simulink library "bcm"  (R2021b)
settings: Solver=VariableStepAuto  StartTime=0.0  StopTime=10.0  RelTol=1e-3
undefined symbols (not defined in the file or in its folder): ENUM_ANTITHEFT_ALARM, ENUM_ANTITHEFT_ARM, ENUM_ANTITHEFT_DISARM, ENUM_ANTITHEFT_WAIT, ENUM_GEARPOSNTOCAN_P, ENUM_PDKEYRAWLULOCK_INUNLOCK, ENUM_PDKEYRAWPS_INPS, ENUM_POWERSTA_ON, ENUM_POWERSTA_READY, ENUM_POWERSTA_STANDBY, ENUM_PWRSTASW_ON, ENUM_PWRSTASW_READY, ENUM_VEHICLETYPE_D21, ENUM_VEHICLETYPE_D31F25, ENUM_VEHICLETYPE_D31HAWD, ENUM_VEHICLETYPE_D31HRWD, ENUM_VEHICLETYPE_D31L24, FALSE, KBCM_ACCSwcPrsTmr_s, KBCM_ALMBrightnessDark_enum, KBCM_AmbBlue_enum, KBCM_AmbBreathT_ms, KBCM_AmbGreen_enum, KBCM_AmbMidPple_enum, KBCM_AmbRed_enum, KBCM_AmbTempCtrlEN_flg, KBCM_AmbTempT_s, KBCM_AmbWelModeENWait_s, KBCM_Antitheft_enum_ovrdflg, KBCM_Antitheft_enum_ovrdval, KBCM_APMDoorCtrlSta_flg_ovrdflg, KBCM_APMDoorCtrlSta_flg_ovrdval, KBCM_CmdKeepT_s, KBCM_CSWLightRstDebT_s, KBCM_CSWTurnLPRstT_s, KBCM_DelayTSW_flg, KBCM_DiagDRLOFF_flg, KBCM_DiagFLTC_mA, KBCM_DiagFMHT_s, KBCM_DiagFRTC_mA, KBCM_DiagRLTC_mA, KBCM_DiagRRTC_mA, KBCM_DrAPMRetryTimes_cnt, KBCM_DrOpenWdwOT_s, KBCM_DrOpenWdwReady_s, KBCM_ESSOffT_ms, KBCM_ESSOnT_ms, KBCM_FDCDKCReDetectT_K, KBCM_FDCDKCUSSFilterT_K, KBCM_HandleLampKeepT_s, KBCM_IVIRstHoldT_ms, KBCM_IVIRstTriggerT_ms, KBCM_ONDelayT_ms, KBCM_RAPSAbnFlashOFFT_ms, KBCM_RAPSAbnFlashONT_ms, KBCM_ReDetectT_K, KBCM_RightHandDriveEN_flg, KBCM_RLSLowSpdFilterT_s, KBCM_RmLampKeep_min, KBCM_RmLpKeyInT_s ... (+37)
libraries: simulink x447, $bdroot x11, hcu_lib x2
(part 12 of 13)

== stateflow chart bcm/BCM/BCM/CenterDoorLock/Chart ==
  settings: updateMethod=DISCRETE
  state CrashDetect [parallel]
    settings: executionOrder=7
    state OFF [commented out]
    state KeyON [commented out]
      state Initial [commented out]
        en:
        CrashDetd=0;
      state sCrash [commented out]
        en:CrashDetd=1;Unlockreq=1;
      note: 750 ms
      state Detect [commented out]
      Initial -> Detect [commented out] : [after(75,tick)]
      Detect -> sCrash [commented out] : [CrashOutputSts>0||....
          | (CrashInputFreq>4.1&&....
          | CrashInputFreq<4.2&&....
          | CrashInputDuty>16&&....
          | CrashInputDuty<17)]
    (default) -> CrashDetect.OFF [commented out]
    CrashDetect.OFF -> Initial [commented out] : [PwrSta>3]
    KeyON -> CrashDetect.OFF [commented out] : [PwrSta<=3]
    (default) -> (junction 1980)
    (junction 1980) -> (junction 1981) : [hasChanged(CrashDetd) && CrashDetd == TRUE]
    CrashDetect -> (junction 1980)
    (junction 1981) -> (junction 1979) : {Unlockreq=1;}
  state ChargingDoor [parallel]
    settings: executionOrder=1
    state ChargingDoorUnlock
      en:FrChargingDoorCtrl=0;
      RrChargingDoorCtrl=0;
      FuelDoorPos=0;
    state U2L
      en:FrChargingDoorCtrl=2;
      RrChargingDoorCtrl=2;
    note: 100ms
    note: 100ms
    state L2U
      en:FrChargingDoorCtrl=1;
      RrChargingDoorCtrl=1;
    state ChargingDoorLock
      en:FrChargingDoorCtrl=0;
      RrChargingDoorCtrl=0;
      FuelDoorPos=1;
    (default) -> (junction 1986)
    (junction 1986) -> (junction 1988) [order 2]
    (junction 1986) -> ChargingDoorUnlock [order 1] : [!EEP_FuelDoorPos]
    (junction 1988) -> ChargingDoorLock
    ChargingDoorUnlock -> U2L : [AntitheftSta==1||AntitheftSta==3]
    L2U -> ChargingDoorUnlock : [after(10,tick)]
    U2L -> ChargingDoorLock : [after(10,tick)]
    ChargingDoorLock -> L2U : [AntitheftSta==0||AntitheftSta==2]
  state IVICentralDoorLockSW [parallel]
    settings: executionOrder=3
    state Release
    state Press
    (default) -> IVICentralDoorLockSW.Press
    IVICentralDoorLockSW.Press -> IVICentralDoorLockSW.Release : [CDL_Unlock_Butt==0&&CDL_Lock_Butt==0]
    IVICentralDoorLockSW.Release -> (junction 1950) [order 1] : [CDL_Lock_Butt==1]
    (junction 1950) -> IVICentralDoorLockSW.Press [order 1] : [BCM_DoorLock_Sta]/{Main.eDUnlock;}
    (junction 1950) -> (junction 1951) [order 2]
    (junction 1951) -> IVICentralDoorLockSW.Press [order 1] : [AllDoorSW]/{Main.eDUnlock;}
    (junction 1951) -> (junction 1952) [order 2]
    (junction 1952) -> IVICentralDoorLockSW.Press [order 1] : [CrashDetd==1]{Main.eDUnlock;}
    (junction 1952) -> (junction 1953) [order 2]
    (junction 1953) -> IVICentralDoorLockSW.Press : {Main.eCTDLock;}
    IVICentralDoorLockSW.Release -> IVICentralDoorLockSW.Press [order 2] : [CDL_Unlock_Butt==1]{Main.eDUnlock;}
  state ATLockCtrl [parallel]
    settings: executionOrder=4
    state LockSend
      en:
      fUnlockSingle=1;
    state NoCommand
    state UnlockSend
      en:fUnlockSingle=0;
    (default) -> NoCommand : {fUnlockSingle=VINP_FlashfUnlockSingle_flg;}
    NoCommand -> (junction 1862) [order 2] : [ATLockCtrl==1]
    (junction 1862) -> LockSend [order 1] : [CrashDetd==1]
    (junction 1862) -> (junction 1865) [order 2] : {Main.eDLock;}
    (junction 1865) -> LockSend [order 1] : [LockSetting]
    (junction 1865) -> (junction 1867) [order 2]
    (junction 1867) -> LockSend
    LockSend -> NoCommand : [ATLockCtrl!=1]
    NoCommand -> (junction 1870) [order 1] : [ATLockCtrl==2....
        | ||....
        | VBCM_AutoUnlockReq_flg]
    (junction 1870) -> UnlockSend [order 1] : [LockSetting==0||fUnlockSingle==0]/{Main.eDUnlock;}
    (junction 1870) -> (junction 1872) [order 2]
    (junction 1872) -> UnlockSend : /{Main.eSUnlock;}
    UnlockSend -> NoCommand : [ATLockCtrl!=2 && !VBCM_AutoUnlockReq_flg]
  state CentralDoorLockSW [parallel]
    settings: executionOrder=2
    state Release
    state Press
    (default) -> CentralDoorLockSW.Press
    CentralDoorLockSW.Press -> CentralDoorLockSW.Release : [!CentralDoorLockSW]
    CentralDoorLockSW.Release -> (junction 1817) : [CentralDoorLockSW]
    (junction 1817) -> CentralDoorLockSW.Press [order 1] : [BCM_DoorLock_Sta]/{Main.eDUnlock;}
    (junction 1817) -> (junction 1821) [order 2]
    (junction 1821) -> CentralDoorLockSW.Press [order 1] : [AllDoorSW]/{Main.eDUnlock;}
    (junction 1821) -> (junction 1824) [order 2]
    (junction 1824) -> CentralDoorLockSW.Press [order 1] : [CrashDetd==1]{Main.eDUnlock;}
    (junction 1824) -> (junction 1827) [order 2]
    (junction 1827) -> CentralDoorLockSW.Press : {Main.eCTDLock;}
  state AutoFoldforHandle [parallel]
    settings: executionOrder=10
    state sStop
    state sMoving
    (default) -> sStop
    sMoving -> sStop : [VehSpeed <= 0]
    sStop -> (junction 2026) : [VehSpeed >= 10 && VehSpeed < 256]
    (junction 2026) -> sMoving [order 1] : [!CrashDetd && ...
        | (!VINP_FLHandleClose_flg || !VINP_FRHandleClose_flg || ....
        |  !VINP_RLHandleClose_flg || !VINP_RRHandleClose_flg)]
        | {VBCM_FDHandleCmd_enum = 3;
        |  LHandleLampCtrl = 1;
        |  RHandleLampCtrl = 1;}
    (junction 2026) -> (junction 2027) [order 2]
    (junction 2027) -> sMoving
  state LED [parallel]
    settings: executionOrder=6
    state OFF
      en:DoorLockIND=0;
    state ON
      en:DoorLockIND=1;
    note: 10 sec
    state HoldON
      en:DoorLockIND=1;
    (default) -> LED.OFF
    ON -> LED.OFF [order 1] : [BCM_DoorLock_Sta==0]
    LED.OFF -> ON [order 1] : [PwrSta>3&&BCM_DoorLock_Sta==1]
    HoldON -> LED.OFF [order 1] : [after(1000,tick)||BCM_DoorLock_Sta==0]
    LED.OFF -> HoldON [order 2] : eResetLED[BCM_DoorLock_Sta==1]
    HoldON -> ON [order 2] : [PwrSta>3]
    ON -> HoldON [order 2] : [PwrSta<=3]
    HoldON -> HoldON [order 3] : eResetLED
  state Main [parallel]
    settings: executionOrder=5
    note: 350 ms
    state WaitForReverse
      en:CTDCtrl=0;
    state StandBy
      en:CTDCtrl=0;
    state DoorLock
      en:CTDCtrl=3;
    note: 100 ms
    state DrDoorUnlock
      en:CTDCtrl=1;
      fVIGHandle=0;
    note: Unlockreq
    state DoorUnlock
      en:CTDCtrl=2;
      fVIGHandle=0;
      ex:Unlockreq=0;
    (default) -> Main.StandBy
    Main.StandBy -> DoorLock [order 1] : eDLock
    DoorLock -> WaitForReverse [order 1] : [after(35,tick)]/{LED.eResetLED;}
    DoorLock -> WaitForReverse [order 2] : [Unlockreq]/{LED.eResetLED;}
    Main.StandBy -> DoorLock [order 5] : eCTDLock{fVIGHandle=1;}
    WaitForReverse -> Main.StandBy : [after(10,tick)]
    Main.StandBy -> DrDoorUnlock [order 2] : eSUnlock
    DrDoorUnlock -> WaitForReverse [order 1] : [after(35,tick)]
    DrDoorUnlock -> DoorUnlock [order 2] : eDUnlock
    DrDoorUnlock -> DoorUnlock [order 3] : [Unlockreq]
    DoorUnlock -> WaitForReverse : [after(35,tick)]
    Main.StandBy -> DoorUnlock [order 3] : eDUnlock
    Main.StandBy -> DoorUnlock [order 4] : [Unlockreq]
  state LHandleLampPowerCtrlforHandle [parallel]
    settings: executionOrder=12
    state sKeep
      en:
      VBCM_FDLHandleLampCmd_flg = 1;
    state sStandBy
      en:
      VBCM_FDLHandleLampCmd_flg = 0;
      LHandleLampCtrl = 0;
    LHandleLampPowerCtrlforHandle -> LHandleLampPowerCtrlforHandle.sKeep : [hasChanged(VBCM_FDHandleCmd_enum) && ...
        | (VBCM_FDHandleCmd_enum == 1 || ...
        |  VBCM_FDHandleCmd_enum == 2)]
    LHandleLampPowerCtrlforHandle.sKeep -> LHandleLampPowerCtrlforHandle.sStandBy : [after (KBCM_HandleLampKeepT_s, tick) || ...
        | (LHandleLampCtrl && ...
        |  VINP_FLHandleClose_flg)]
    (default) -> LHandleLampPowerCtrlforHandle.sStandBy
  state DoorOpenDetectforHandle [parallel]
    settings: executionOrder=8
    state sDrDoorOpenDet [parallel]
      settings: executionOrder=1
      (default) -> (junction 2039)
      sDrDoorOpenDet -> (junction 2038) : [hasChanged(VINP_DrDoorSW_flg) && VINP_DrDoorSW_flg]
      (junction 2038) -> (junction 2039) : [VehSpeed <= 0 && VINP_FLHandleClose_flg]
          | {VBCM_FDHandleCmd_enum = 1;
          |  LHandleLampCtrl = 0;}
    state sPsDoorOpenDet [parallel]
      settings: executionOrder=2
      (default) -> (junction 2045)
      (junction 2044) -> (junction 2045) : [VehSpeed <= 0 && ...
          | (VINP_FLHandleClose_flg || VINP_FRHandleClose_flg)]
          | {VBCM_FDHandleCmd_enum = 2;
          |  RHandleLampCtrl = 0;}
      sPsDoorOpenDet -> (junction 2044) : [hasChanged(VINP_PsDoorSW_flg) && VINP_PsDoorSW_flg]
    state sRLDoorOpenDet [parallel]
      settings: executionOrder=3
      (default) -> (junction 2051)
      sRLDoorOpenDet -> (junction 2050) : [hasChanged(VINP_RLDoorSW_flg) && VINP_RLDoorSW_flg]
      (junction 2050) -> (junction 2051) : [VehSpeed <= 0 && ...
          | (VINP_FLHandleClose_flg || VINP_RLHandleClose_flg)]
          | {VBCM_FDHandleCmd_enum = 2;
          |  RHandleLampCtrl = 0;}
    state sRRDoorOpenDet [parallel]
      settings: executionOrder=4
      (default) -> (junction 2057)
      sRRDoorOpenDet -> (junction 2056) : [hasChanged(VINP_RRDoorSW_flg) && VINP_RRDoorSW_flg]
      (junction 2056) -> (junction 2057) : [VehSpeed <= 0 && ...
          | (VINP_FLHandleClose_flg || VINP_RRHandleClose_flg)]
          | {VBCM_FDHandleCmd_enum = 2;
          |  RHandleLampCtrl = 0;}
  state AutoLock [parallel]
    settings: executionOrder=14
    state StandBy
      en:
      VBCM_AutoUnlockReq_flg = 0;
    state AutoLock
      en:
      Main.eDLock;
      VBCM_AutoLockDisable_flg = 1;
    state AutoUnlock
      en:
      VBCM_AutoUnlockReq_flg = 1;
      VBCM_AutoLockDisable_flg = 0;
    state AutoLockENRst
      en:
      VBCM_AutoLockDisable_flg = 0;
    (default) -> AutoLock.StandBy
    AutoLock.StandBy -> AutoLock.AutoLock [order 3] : [AirBagFailCmd==0 && CrashDetd==0 && VehSpeed>=10 && VBCM_AutoLockSta_flg && !VBCM_AutoLockDisable_flg]
    AutoLock.AutoLock -> AutoLock.StandBy
    AutoLock.StandBy -> AutoUnlock [order 1] : [VBCM_AutoUnlockSta_flg && ShiftGearPosnBuf != 0 && VTQD_ShiftGearPosn_enum == 0]
    AutoUnlock -> AutoLock.StandBy
    AutoLock.StandBy -> AutoLockENRst [order 2] : [(hasChanged(AllDoorSW) && AllDoorSW == 1)....
        | ||....
        | (PwrStaBuf == 4 || PwrStaBuf == 5) && (PwrSta >= 0 && PwrSta <= 3)....
        | ||....
        | (hasChanged(VBCM_AutoLockSta_flg) && VBCM_AutoLockSta_flg)]
    AutoLockENRst -> AutoLock.StandBy
  state RHandleLampPowerCtrlforHandle [parallel]
    settings: executionOrder=13
    state sKeep
      en:
      VBCM_FDRHandleLampCmd_flg = 1;
    state sStandBy
      en:
      VBCM_FDRHandleLampCmd_flg = 0;
      RHandleLampCtrl = 0;
    RHandleLampPowerCtrlforHandle -> RHandleLampPowerCtrlforHandle.sKeep : [hasChanged(VBCM_FDHandleCmd_enum) && ....
        | VBCM_FDHandleCmd_enum == 2]
    RHandleLampPowerCtrlforHandle.sKeep -> RHandleLampPowerCtrlforHandle.sStandBy : [after (KBCM_HandleLampKeepT_s, tick) || ...
        | (RHandleLampCtrl && ...
        |  VINP_FRHandleClose_flg &&....
        |  VINP_RLHandleClose_flg &&....
        |  VINP_RRHandleClose_flg)]
    (default) -> RHandleLampPowerCtrlforHandle.sStandBy
  state CmdReset [parallel]
    settings: executionOrder=11
    state sKeep
    state sStandBy
      en:
      VBCM_FDHandleCmd_enum = 0;
    CmdReset -> CmdReset.sKeep : [hasChanged(VBCM_FDHandleCmd_enum) && ...
        | VBCM_FDHandleCmd_enum > 0]
    CmdReset.sKeep -> CmdReset.sStandBy : [after (KBCM_CmdKeepT_s, tick)]
    (default) -> CmdReset.sStandBy
  state CTDDoorCtrlforHandle [parallel]
    settings: executionOrder=9
    (default) -> (junction 2009)
    (junction 2008) -> (junction 2009) [order 1] : [VehSpeed <= 0 && CTDCtrl == 1]
        | {VBCM_FDHandleCmd_enum = CTDCtrl;
        |  LHandleLampCtrl = 0;}
    CTDDoorCtrlforHandle -> (junction 2008) : [hasChanged(CTDCtrl) && CTDCtrl > 0]
    (junction 2008) -> (junction 2010) [order 2]
    (junction 2010) -> (junction 2011) [order 1] : [VehSpeed <= 0 && CTDCtrl == 2]
        | {VBCM_FDHandleCmd_enum = CTDCtrl;
        |  LHandleLampCtrl = 0;
        |  RHandleLampCtrl = 0;}
    (junction 2010) -> (junction 2012) [order 2] : [VehSpeed <= 0 && CTDCtrl == 3]
        | {VBCM_FDHandleCmd_enum = CTDCtrl;
        |  LHandleLampCtrl = 1;
        |  RHandleLampCtrl = 1;}
  data: AntitheftSta input uint8 [..3]; FrChargingDoorCtrl output uint8 [0..2]; RrChargingDoorCtrl output uint8 [0..2]; AllDoorSW input boolean; PwrSta input uint8 [0..5]; CentralDoorLockSW input boolean; BCM_DoorLock_Sta input boolean; CTDCtrl output uint8 [0..3]; DoorLockIND output boolean; ATLockCtrl input uint8 [0..2]; AirBagFailCmd input boolean; VehSpeed input; fVIGHandle output boolean; CDL_Unlock_Butt input boolean; CDL_Lock_Butt input boolean; Unlockreq local boolean; CrashDetd input boolean; FuelDoorPos output; EEP_FuelDoorPos input; fUnlockSingle output boolean; VINP_FlashfUnlockSingle_flg input; KBCM_CmdKeepT_s input; KBCM_HandleLampKeepT_s input; VINP_DrDoorSW_flg input; VINP_FLHandleClose_flg input; VINP_FRHandleClose_flg input; VINP_PsDoorSW_flg input; VINP_RLDoorSW_flg input; VINP_RLHandleClose_flg input; VINP_RRDoorSW_flg input; VINP_RRHandleClose_flg input; VBCM_FDLHandleLampCmd_flg output boolean; VBCM_FDRHandleLampCmd_flg output boolean; LHandleLampCtrl local boolean; RHandleLampCtrl local boolean; VBCM_FDHandleCmd_enum output uint8; LockSetting input =0; PwrStaBuf input; ShiftGearPosnBuf input; VBCM_AutoLockSta_flg input; VBCM_AutoUnlockSta_flg input; VTQD_ShiftGearPosn_enum input; VBCM_AutoLockDisable_flg local boolean; VBCM_AutoUnlockReq_flg local boolean; TRUE parameter
  events: eResetLED local FUNCTION_CALL_EVENT; eDLock local FUNCTION_CALL_EVENT; eDUnlock local FUNCTION_CALL_EVENT; eSUnlock local FUNCTION_CALL_EVENT; eCTDLock local FUNCTION_CALL_EVENT

== stateflow chart bcm/BCM/BCM/Dimmer/Chart ==
  settings: sampleTime=StepSize
  state CANDimmerCMD [parallel]
    settings: executionOrder=1
    state sWait
    (default) -> sWait
    (junction 1680) -> sWait : [MFRD_N_Bright_Req<=100&&IVI_Status]/{Dimmer=20+MFRD_N_Bright_Req*0.8}
    (junction 1677) -> (junction 1680) [order 1]
    (junction 1677) -> sWait [order 2]
    (junction 1609) -> (junction 1677)
    sWait -> (junction 1609) : [after(20,tick)]
  state sDimmer_EN [parallel]
    settings: executionOrder=2  description=This state models the modes of a door sensor and implements logic to respond when that sensor is producing a signal.
    state sOFF
      en:DimmerEN=0;
    state sON
      en:DimmerEN=1;
    (default) -> sOFF
      settings: description=On the first sample call the door mode is set to active.
    sON -> sOFF : [!PLamp||IVI_Night_Mode_Sta]
    sOFF -> sON : [PLamp&&!IVI_Night_Mode_Sta]
  data: IVI_Status input boolean; IVI_Night_Mode_Sta input boolean; Dimmer output single =0; DimmerEN output boolean; PLamp input boolean; MFRD_N_Bright_Req input =0
  data IVI_Night_Mode_Sta settings: description=Min=0, Max=2047, Engineering Unit = km/h, Offset=0 km/h, Resolution= 0.125 km/h per bit, >2047 = Invalid (bit 12 = 1)
  data Dimmer settings: description=|
      | Bcm Buzzer output results.
      | 0 = None Buzzer
      | 1 = Turn signal Buzzer
      | 2 = Key Reminder Buzzer
      | 3 = Seat Belt Buzzer
      | 4 = Light Monitor Buzzer

== stateflow chart bcm/BCM/BCM/ExteriorLight/Chart ==
  settings: updateMethod=DISCRETE
  state FollowMeSW [parallel]
    settings: executionOrder=2
    state Disabled
    state Enabled
    (default) -> Disabled
    Disabled -> Enabled : [FDC_BCM_FollowMeENFun_Sta==1]
    Enabled -> (junction 2763) [order 2] : [(VBCM_PwrStaBuf_enum==4 || VBCM_PwrStaBuf_enum==5) &&....
        | (VPMM_PwrSta_enum==1 || VPMM_PwrSta_enum==2)]
        | {AutoCut.eFollow;}
    (junction 2763) -> (junction 2765)
    (junction 2755) -> Disabled [order 1] : [VBCM_FollowMe_flg==1]
        | {AutoCut.eFollow;}
    Enabled -> (junction 2755) [order 1] : [FDC_BCM_FollowMeENFun_Sta==0]
    (junction 2755) -> (junction 2758) [order 2]
    (junction 2765) -> Enabled
    (junction 2758) -> Disabled
  state RFogLamp [parallel]
    settings: executionOrder=1
    state sON
      en:VBCM_RrFogLamp_flg=1;
    state sOFF
      en:VBCM_RrFogLamp_flg=0;
    (default) -> RFogLamp.sOFF
    RFogLamp.sOFF -> RFogLamp.sON : [VPMM_PwrSta_enum>3&&....
        | VINP_RFogLampSW_flg==1&&....
        | VBCM_LBeam_flg==1]
    RFogLamp.sON -> RFogLamp.sOFF : [VPMM_PwrSta_enum<=3||....
        | VINP_RFogLampSW_flg==0||....
        | VBCM_LBeam_flg==0]
  state DRL [parallel]
    settings: executionOrder=3
    state sOFF
      en:VBCM_LDRL_flg=0;
      VBCM_RDRL_flg=0;
    state DRL_Opearting
      state sDebounce
      state sON
        en:VBCM_LDRL_flg=1;
        VBCM_RDRL_flg=1;
      note: 300 ms
      state TurnLeft
        en:VBCM_LDRL_flg=0;
        VBCM_RDRL_flg=1;
      state TurnRight
        en:VBCM_LDRL_flg=1;
        VBCM_RDRL_flg=0;
      sDebounce -> (junction 2687) : [after(30,tick)]
      (junction 2687) -> DRL.DRL_Opearting.sON [order 1] : [VBCM_OutMode_enum==0]
      (junction 2687) -> (junction 2689) [order 2]
      DRL.DRL_Opearting.sON -> TurnLeft [order 1] : [VBCM_OutMode_enum==1]
      TurnLeft -> DRL.DRL_Opearting.sON [order 1] : [VBCM_OutMode_enum==0]
      TurnRight -> DRL.DRL_Opearting.sON [order 2] : [VBCM_OutMode_enum==0]
      DRL.DRL_Opearting.sON -> TurnRight [order 2] : [VBCM_OutMode_enum==2]
      (junction 2689) -> TurnLeft [order 1] : [VBCM_OutMode_enum==1]
      (junction 2689) -> (junction 2701) [order 2]
      TurnRight -> TurnLeft [order 1] : [VBCM_OutMode_enum==1]
      TurnLeft -> TurnRight [order 2] : [VBCM_OutMode_enum==2]
      (junction 2701) -> TurnRight
    (default) -> DRL.sOFF
    DRL.sOFF -> sDebounce : [VBCM_DiagDRLOFF_flg==0 &&...
        | VPMM_PwrSta_enum==ENUM_POWERSTA_READY &&...
        | (VTQD_ShiftGearPosn_enum != ENUM_GEARPOSNTOCAN_P || VINP_HeadLampSW_enum==0) &&...
        | !VBCM_PosLamp_flg &&...
        | VBCM_OutMode_enum < 3]
    DRL_Opearting -> DRL.sOFF : [VBCM_DiagDRLOFF_flg==1 ||...
        | VPMM_PwrSta_enum!=ENUM_POWERSTA_READY ||...
        | (VTQD_ShiftGearPosn_enum == ENUM_GEARPOSNTOCAN_P && VINP_HeadLampSW_enum!=0) ||...
        | VBCM_PosLamp_flg ||...
        | VBCM_OutMode_enum >= 3]
  state sBrakeLamp [parallel]
    settings: executionOrder=4
    state sON
      en:VBCM_BrakeLamp_flg=1;
    state sOFF
      en:VBCM_BrakeLamp_flg=0;
    (default) -> sBrakeLamp.sOFF
    sBrakeLamp.sOFF -> sBrakeLamp.sON : [VINP_BrakeSWGPIO_flg==1 || VTQD_ReBrakeLPReq_flg==1 || VINP_ActBrkLampSta_flg==1]
    sBrakeLamp.sON -> sBrakeLamp.sOFF : [VINP_BrakeSWGPIO_flg==0 && VTQD_ReBrakeLPReq_flg==0 && VINP_ActBrkLampSta_flg==0]
  state sReverseLamp [parallel]
    settings: executionOrder=5
    state sON
      en:VBCM_ReverseLamp_flg=1;
    state sOFF
      en:VBCM_ReverseLamp_flg=0;
    (default) -> sReverseLamp.sOFF
    sReverseLamp.sOFF -> sReverseLamp.sON : [VPMM_PwrSta_enum>3&&VTQD_ShiftGearPosn_enum==7]
    sReverseLamp.sON -> sReverseLamp.sOFF : [VPMM_PwrSta_enum<=3||VTQD_ShiftGearPosn_enum!=7]
  state sATCtrl [parallel]
    settings: executionOrder=6
    state StandBy
    state Lock
      en:send(AutoCut.eLock);
    state Unlock
      en:send(AutoCut.eUnlock);
    (default) -> StandBy
    StandBy -> Lock [order 1] : [VBCM_ATCtrl_enum==1]
    Lock -> StandBy : [VBCM_ATCtrl_enum!=1]
    StandBy -> sATCtrl.Unlock [order 2] : [VBCM_ATCtrl_enum==2]
    sATCtrl.Unlock -> StandBy : [VBCM_ATCtrl_enum!=2]
  state PositionLamp [parallel]
    settings: executionOrder=11
    state sPositionLamp
      en:VBCM_PosLamp_flg=1;
    state sOFF
      en:VBCM_PosLamp_flg=0;
    (default) -> PositionLamp.sOFF
    (junction 2636) -> sPositionLamp [order 1] : [VINP_HeadLampSW_enum==1||VINP_HeadLampSW_enum==2]
    PositionLamp.sOFF -> (junction 2636) [order 1] : [!VBCM_AutoCut_flg]
    (junction 2636) -> (junction 2637) [order 2]
    (junction 2637) -> sPositionLamp [order 1] : [VPMM_PwrSta_enum > 3 &&....
        | VINP_HeadLampSW_enum == 0 &&....
        | VINP_RLSLampSta_flg]
    (junction 2637) -> (junction 2638) [order 2]
    (junction 2638) -> sPositionLamp : [VBCM_FollowMe_flg]
    PositionLamp.sOFF -> sPositionLamp [order 2] : [VBCM_showupEN_flg && VBCM_showup_flg]
    (junction 2639) -> PositionLamp.sOFF : [!VBCM_FollowMe_flg &&....
        | (VINP_HeadLampSW_enum == 3 ||....
        | (VINP_HeadLampSW_enum == 0 &&....
        | (VPMM_PwrSta_enum <= 3 || !VINP_RLSLampSta_flg)))]
    (junction 2640) -> (junction 2639) [order 2]
    (junction 2640) -> PositionLamp.sOFF [order 1] : [VBCM_AutoCut_flg]
    sPositionLamp -> (junction 2640) : [!VBCM_showupEN_flg || !VBCM_showup_flg]
  state AutoCut [parallel]
    settings: executionOrder=12
    state FollowMeHome
      en:
      VBCM_FollowMe_flg=1;
      VBCM_AutoCut_flg=0;
      VBCM_showup_flg=0;
      ex:
      VBCM_FollowMe_flg=0;
    state Normal
      state sNormal
        en:VBCM_AutoCut_flg=0;
        VBCM_showup_flg=0;
      state AutoCutDetect
      note: 40 sec
      state Unlock
        en:VBCM_AutoCut_flg=1;
        VBCM_showup_flg=1;
        note: 30 sec
      state AutoCut
        en:VBCM_AutoCut_flg=1;
        VBCM_showup_flg=0;
        VBCM_FollowMe_flg=0;
      sNormal -> AutoCutDetect : [VPMM_PwrSta_enum<=3&&(VINP_HeadLampSW_enum!=3)]
      (junction 2665) -> sNormal : [VPMM_PwrSta_enum>3||VINP_HeadLampSW_enum==3]
      AutoCutDetect -> (junction 2665) [order 1]
      AutoCut.Normal.AutoCut -> (junction 2665)
      AutoCutDetect -> AutoCut.Normal.AutoCut [order 2] : eLock
      AutoCutDetect -> AutoCut.Normal.AutoCut [order 3] : [after(4000,tick)]
      AutoCut.Normal.Unlock -> sNormal [order 2] : [VPMM_PwrSta_enum>3]
      (default) -> AutoCut.Normal.AutoCut
      AutoCut.Normal.Unlock -> AutoCut.Normal.AutoCut [order 1] : eLock
      AutoCut.Normal.Unlock -> AutoCut.Normal.AutoCut [order 3] : [after(3000,tick)]
      Normal -> AutoCut.Normal.Unlock [order 1] : eUnlock[VPMM_PwrSta_enum<=3]
    note: 4000
    note: 40 sec
    (default) -> Normal
    Normal -> FollowMeHome [order 1] : eFollow[VPMM_PwrSta_enum<=3]
    FollowMeHome -> sNormal [order 2] : eFollow
    FollowMeHome -> sNormal [order 3] : [VPMM_PwrSta_enum>3]
    FollowMeHome -> (junction 2717) [order 1] : [after(VBCM_DiagFMHT_s,tick)]
    (junction 2717) -> sNormal [order 1] : [VPMM_PwrSta_enum>3||...
        |  VINP_HeadLampSW_enum==3]
    (junction 2717) -> (junction 2719) [order 2]
    (junction 2719) -> AutoCut.Normal.AutoCut
  state LowBeam [parallel]
    settings: executionOrder=8
    state sLBeam
      en:VBCM_LBeam_flg=1;
    state sOFF
      en:VBCM_LBeam_flg=0;
    (default) -> LowBeam.sOFF
    (junction 2417) -> sLBeam [order 1] : [VBCM_HBeam_flg]
    LowBeam.sOFF -> (junction 2417) [order 1] : [!VBCM_AutoCut_flg]
    (junction 2417) -> (junction 2418) [order 2]
    (junction 2418) -> sLBeam [order 1] : [VINP_HeadLampSW_enum==2]
    (junction 2418) -> (junction 2419) [order 2]
    (junction 2419) -> sLBeam [order 1] : [VPMM_PwrSta_enum > VBCM_HLBeamENPwrSta_enum &&....
        | VINP_HeadLampSW_enum == 0 &&....
        | VINP_RLSLampSta_flg]
    (junction 2419) -> (junction 2420) [order 2]
    (junction 2420) -> sLBeam : [VBCM_FollowMe_flg]
    LowBeam.sOFF -> sLBeam [order 2] : [VBCM_showupEN_flg && VBCM_showup_flg]
    (junction 2421) -> LowBeam.sOFF [order 1] : [VBCM_AutoCut_flg]
    sLBeam -> (junction 2421) : [!VBCM_showupEN_flg || !VBCM_showup_flg]
    (junction 2421) -> (junction 2422) [order 2]
    (junction 2422) -> LowBeam.sOFF : [!VBCM_FollowMe_flg &&....
        | !VBCM_HBeam_flg &&....
        | VINP_HeadLampSW_enum != 2 &&....
        | (VINP_HeadLampSW_enum!=0 ||....
        | !VINP_RLSLampSta_flg ||....
        | VPMM_PwrSta_enum <= VBCM_HLBeamENPwrSta_enum)]
  state HighBeam [parallel]
    settings: executionOrder=7
    state sOFF
      en:VBCM_HBeam_flg=0;
    state sHBeam
      en:VBCM_HBeam_flg=1;
    (default) -> HighBeam.sOFF
    HighBeam.sOFF -> (junction 2455) : [!VBCM_AutoCut_flg]
    (junction 2455) -> HighBeam.sHBeam [order 1] : [VINP_CSWPassSWSta_flg]
    (junction 2455) -> (junction 2456) [order 2]
    (junction 2456) -> (junction 2457) : [VINP_CSWDimSw_flg]
    (junction 2457) -> HighBeam.sHBeam [order 1] : [VINP_HeadLampSW_enum==2]
    (junction 2457) -> (junction 2458) [order 2]
    (junction 2458) -> HighBeam.sHBeam : [VINP_HeadLampSW_enum == 0 &&....
        | VINP_RLSLampSta_flg == 1 &&....
        | VINP_ForceLowBeam_enum == 0 &&....
        | VPMM_PwrSta_enum > VBCM_HLBeamENPwrSta_enum &&....
        | VBCM_AutoHLB_flg]
    HighBeam.sHBeam -> HighBeam.sOFF [order 1] : [VBCM_AutoCut_flg]
    HighBeam.sHBeam -> (junction 2459) [order 2] : [!VINP_CSWPassSWSta_flg]
    (junction 2459) -> HighBeam.sOFF [order 1] : [!VINP_CSWDimSw_flg]
    (junction 2459) -> (junction 2605) [order 2]
    (junction 2605) -> (junction 2460) : [VINP_HeadLampSW_enum!=2]
    (junction 2460) -> HighBeam.sOFF [order 1] : [VINP_HeadLampSW_enum!=0]
    (junction 2460) -> (junction 2462) [order 2]
    (junction 2462) -> HighBeam.sOFF [order 1] : [VINP_RLSLampSta_flg==0 || VPMM_PwrSta_enum <= VBCM_HLBeamENPwrSta_enum]
    (junction 2462) -> (junction 2463) [order 2]
    (junction 2463) -> HighBeam.sOFF : [VINP_ForceLowBeam_enum==1||!VBCM_AutoHLB_flg]
  state AutoHLB [parallel]
    settings: executionOrder=13
    state AutoON
      on after(KBCM_ONDelayT_ms, tick):
      VBCM_AutoHLB_flg = TRUE;
    state AutoOFF
      en:
      VBCM_AutoHLB_flg = FALSE;
    (default) -> AutoOFF
    AutoOFF -> AutoON : [VINP_METERKPHCalcu_kph >= 30]
    AutoON -> AutoOFF : [VINP_METERKPHCalcu_kph <= 25]
  state RBSD_CTRL [parallel]
    settings: executionOrder=10
    state OFF
      en:VBCM_RBSD_flg=0;
    state FlashOFF
      en:VBCM_RBSD_flg=0;
    state ON
      en:VBCM_RBSD_flg=1;
    (default) -> RBSD_CTRL.OFF
    RBSD_CTRL.FlashOFF -> RBSD_CTRL.OFF [order 1] : [VINP_SRRBSDWarnR_enum==0 && VINP_SRRODAWarnR_enum==0]
    RBSD_CTRL.ON -> RBSD_CTRL.FlashOFF [order 2] : [after(13,tick)&&(VINP_SRRBSDWarnR_enum==2||VINP_SRRODAWarnR_enum==2)]
    RBSD_CTRL.FlashOFF -> RBSD_CTRL.ON [order 2] : [after(12,tick)]
    RBSD_CTRL.ON -> RBSD_CTRL.OFF [order 1] : [VINP_SRRBSDWarnR_enum==0 && VINP_SRRODAWarnR_enum==0]
    RBSD_CTRL.OFF -> RBSD_CTRL.ON : [VINP_SRRBSDWarnR_enum>0 || VINP_SRRODAWarnR_enum>0]
  state LBSD_CTRL [parallel]
    settings: executionOrder=9
    state OFF
      en:VBCM_LBSD_flg=0;
    state FlashOFF
      en:VBCM_LBSD_flg=0;
    state ON
      en:VBCM_LBSD_flg=1;
    (default) -> LBSD_CTRL.OFF
    LBSD_CTRL.FlashOFF -> LBSD_CTRL.OFF [order 1] : [VINP_SRRBSDWarnL_enum==0 && VINP_SRRODAWarnL_enum==0]
    LBSD_CTRL.ON -> LBSD_CTRL.FlashOFF [order 2] : [after(13,tick)&&(VINP_SRRBSDWarnL_enum==2||VINP_SRRODAWarnL_enum==2)]
    LBSD_CTRL.FlashOFF -> LBSD_CTRL.ON [order 2] : [after(12,tick)]
    LBSD_CTRL.ON -> LBSD_CTRL.OFF [order 1] : [VINP_SRRBSDWarnL_enum==0 && VINP_SRRODAWarnL_enum==0]
    LBSD_CTRL.OFF -> LBSD_CTRL.ON : [VINP_SRRBSDWarnL_enum>0 || VINP_SRRODAWarnL_enum>0]
  state HighBeam_ADB [parallel]
    settings: executionOrder=14
    state sHBeam
      en:VBCM_HBeamADB_flg=1;
    state sOFF
      en:VBCM_HBeamADB_flg=0;
    (default) -> HighBeam_ADB.sOFF
    (junction 2723) -> HighBeam_ADB.sHBeam [order 1] : [VINP_CSWPassSWSta_flg]
    HighBeam_ADB.sOFF -> (junction 2723) : [!VBCM_AutoCut_flg]
    (junction 2723) -> (junction 2724) [order 2]
    (junction 2725) -> HighBeam_ADB.sHBeam [order 1] : [VINP_HeadLampSW_enum==2]
    (junction 2724) -> (junction 2725) : [VINP_CSWDimSw_flg]
    (junction 2725) -> (junction 2726) [order 2]
    (junction 2726) -> HighBeam_ADB.sHBeam : [VINP_HeadLampSW_enum == 0 &&....
        | VINP_RLSLampSta_flg == 1 &&....
        | VPMM_PwrSta_enum > VBCM_HLBeamENPwrSta_enum]
    HighBeam_ADB.sHBeam -> HighBeam_ADB.sOFF [order 1] : [VBCM_AutoCut_flg]
    (junction 2727) -> HighBeam_ADB.sOFF [order 1] : [!VINP_CSWDimSw_flg]
    HighBeam_ADB.sHBeam -> (junction 2727) [order 2] : [!VINP_CSWPassSWSta_flg]
    (junction 2727) -> (junction 2729) [order 2]
    (junction 2728) -> HighBeam_ADB.sOFF [order 1] : [VINP_HeadLampSW_enum!=0]
    (junction 2729) -> (junction 2728) : [VINP_HeadLampSW_enum!=2]
    (junction 2728) -> (junction 2730) [order 2]
    (junction 2730) -> HighBeam_ADB.sOFF : [VINP_RLSLampSta_flg == 0 ||....
        | VPMM_PwrSta_enum <= VBCM_HLBeamENPwrSta_enum]
  data: VPMM_PwrSta_enum input uint8 [0..5]; VBCM_PwrStaBuf_enum input uint8; VINP_HeadLampSW_enum input uint8 [0..3]; VINP_RFogLampSW_flg input boolean; VINP_BrakeSWGPIO_flg input boolean; VINP_CSWDimSw_flg input boolean; VINP_CSWPassSWSta_flg input boolean; VTQD_ShiftGearPosn_enum input uint8 [0..15]; VBCM_PosLamp_flg output boolean; VBCM_LBeam_flg output boolean; VBCM_HBeam_flg output boolean; VBCM_RrFogLamp_flg output boolean; VBCM_BrakeLamp_flg output boolean; VBCM_ReverseLamp_flg output boolean; VBCM_OutMode_enum input uint8 [0..15]; VBCM_AutoCut_flg local boolean; VBCM_LDRL_flg output boolean; VBCM_RDRL_flg output boolean; VBCM_ATCtrl_enum input uint8 [0..2]; VINP_RLSLampSta_flg input boolean; VINP_ActBrkLampSta_flg input boolean; VINP_SRRODAWarnR_enum input; VINP_SRRODAWarnL_enum input; VINP_SRRBSDWarnR_enum input; VINP_SRRBSDWarnL_enum input; VINP_ForceLowBeam_enum input uint8; VTQD_ReBrakeLPReq_flg input; VBCM_LBSD_flg output boolean; VBCM_RBSD_flg output boolean; VBCM_DiagDRLOFF_flg input; VBCM_DiagFMHT_s input; ENUM_GEARPOSNTOCAN_P parameter; ENUM_POWERSTA_READY parameter; VBCM_showup_flg output boolean; VBCM_AutoHLB_flg local boolean =0; VINP_METERKPHCalcu_kph input; KBCM_ONDelayT_ms input; VBCM_HLBeamENPwrSta_enum input; VBCM_showupEN_flg input; VBCM_FollowMe_flg output boolean; TRUE parameter; FALSE parameter; VBCM_HBeamADB_flg output boolean; FDC_BCM_FollowMeENFun_Sta input
  events: eLock local FUNCTION_CALL_EVENT; eUnlock local FUNCTION_CALL_EVENT; eFollow local FUNCTION_CALL_EVENT

== stateflow chart bcm/BCM/BCM/FlasherSignal/Chart ==
  settings: updateMethod=DISCRETE
  state sModeSelect [parallel]
    settings: executionOrder=2  description=This state models the modes of a door sensor and implements logic to respond when that sensor is producing a signal.
    state sStandBy
    (default) -> sStandBy
      settings: description=On the first sample call the door mode is set to active.
    sStandBy -> (junction 1892)
    (junction 1893) -> sStandBy
    (junction 1892) -> (junction 1893) [order 1] : [ATAlarm==1]{InputMode=6;}
    (junction 1892) -> (junction 1969) [order 2]
    (junction 1971) -> (junction 1893)
    (junction 1969) -> (junction 1971) [order 1] : [(VINP_VehicleType_enum != ENUM_VEHICLETYPE_D21 && InputMode==4) || ....
        |  InputMode == 5 || InputMode == 9]
    (junction 1969) -> (junction 2027) [order 2]
    (junction 2028) -> (junction 1971)
    (junction 2027) -> (junction 2028) [order 1] : [SPTGDet==1]{InputMode=8;}
    (junction 2027) -> (junction 1871) [order 2]
    (junction 1873) -> (junction 2028)
    (junction 1871) -> (junction 1873) [order 1] : [PwrSta>3&&ESS_Active==1]{InputMode=7;}
    (junction 1871) -> (junction 2201) [order 2]
    (junction 2202) -> (junction 1873)
    (junction 2201) -> (junction 2202) [order 1] : [VINP_RAPSErrWarn_enum==2]{InputMode=3;}
    (junction 2201) -> (junction 2175) [order 2]
    (junction 2177) -> (junction 2202)
    (junction 2175) -> (junction 2177) [order 1] : [PwrSta>3&&RAPSBCMLampCmd==1]{InputMode=1;}
    (junction 2175) -> (junction 2206) [order 2]
    (junction 2207) -> (junction 2177)
    (junction 2206) -> (junction 2207) [order 1] : [PwrSta>3&&RAPSBCMLampCmd==2]{InputMode=2;}
    (junction 2206) -> (junction 2212) [order 2]
    (junction 2213) -> (junction 2207)
    (junction 2212) -> (junction 2213) [order 1] : [VBCM_RAPSAbnFlashReq_flg]{InputMode=12;}
    (junction 2212) -> (junction 1987) [order 2]
    (junction 1989) -> (junction 2213)
    (junction 1987) -> (junction 1989) [order 1] : [ RAPSBCMLampCmd==3] {InputMode=3;}
    (junction 1987) -> (junction 1876) [order 2]
    (junction 1878) -> (junction 1989)
    (junction 1876) -> (junction 1878) [order 1] : [HazardSW==1 || VBCM_PwrErrWarn_flg]{InputMode=3;}
    (junction 1876) -> (junction 2196) [order 2]
    (junction 2197) -> (junction 1878)
    (junction 2196) -> (junction 2197) [order 1] : [PwrSta>3&&CSW_TurnSw_Sta==1]{InputMode=1;}
    (junction 2196) -> (junction 1882) [order 2]
    (junction 1884) -> (junction 2197)
    (junction 1882) -> (junction 1884) [order 1] : [PwrSta>3&&CSW_TurnSw_Sta==2]{InputMode=2;}
    (junction 2014) -> (junction 1884)
    (junction 1882) -> (junction 2013) [order 2]
    (junction 2013) -> (junction 2014) [order 1] : [PwrSta>3&&LeftTurnLightReq==1]{InputMode=1;}
    (junction 2013) -> (junction 2007) [order 2]
    (junction 2009) -> (junction 2014)
    (junction 2007) -> (junction 2009) [order 1] : [PwrSta>3&&RightTurnLightReq==1]{InputMode=2;}
    (junction 2007) -> (junction 2170) [order 2]
    (junction 2171) -> (junction 2009)
    (junction 2170) -> (junction 2171) [order 1] : [InputMode==4]
    (junction 2170) -> (junction 2099) [order 2]
    (junction 2100) -> (junction 2171)
    (junction 2099) -> (junction 2100) [order 1] : [VTPM_TPMSTLCmd_flg]{InputMode=11;}
    (junction 2099) -> (junction 1887) [order 2]
    (junction 1889) -> (junction 2100)
    (junction 1887) -> (junction 1889) : /{InputMode=0;}
  state sPTGReq [parallel]
    settings: executionOrder=5
    state StandBy
    state Twice
      en:InputMode=9;
    state ThreeTimes
      en:InputMode=5;
    (default) -> sPTGReq.StandBy
    sPTGReq.StandBy -> Twice [order 1] : [PTG_RDIL_Sta==1]
    Twice -> sPTGReq.StandBy : [PTG_RDIL_Sta==0]
    sPTGReq.StandBy -> ThreeTimes [order 2] : [PTG_RDIL_Sta==2]
    ThreeTimes -> sPTGReq.StandBy : [PTG_RDIL_Sta==0]
  state HazardSW [parallel]
    settings: executionOrder=1
    state Normal
      state sHAZARDOFF
      state Press
      state sHAZARDON
      (default) -> sHAZARDOFF
      sHAZARDOFF -> Press : [HazardSWSta==1]/{HazardSW=1;}
      (junction 1864) -> sHAZARDOFF [order 1] : [HazardSW==0]
      Press -> (junction 1864) : [HazardSWSta==0]
      (junction 1864) -> sHAZARDON [order 2]
      sHAZARDON -> Press : [HazardSWSta==1]{HazardSW=0;}
    state ADASHazardReq
    (default) -> Normal
    ADASHazardReq -> sHAZARDON : [HazardWarningReq==0]
    Normal -> ADASHazardReq : [HazardWarningReq==1]{HazardSW=1}
  state sATCtrl [parallel]
    settings: executionOrder=4
    state StandBy
    state Lock
      en:InputMode=4;
    state Unlock
      en:InputMode=5;
    (default) -> sATCtrl.StandBy
    sATCtrl.StandBy -> Lock [order 1] : [ATCtrl==1]
    Lock -> sATCtrl.StandBy : [ATCtrl!=1]
    sATCtrl.StandBy -> Unlock [order 2] : [ATCtrl==2]
    Unlock -> sATCtrl.StandBy : [ATCtrl!=2]
  state sPowerErrorWarning [parallel]
    settings: executionOrder=6
    state sWarningOFF
      en:
      VBCM_PwrErrWarn_flg = FALSE;
    state sWarningON
      en:
      VBCM_PwrErrWarn_flg = TRUE;
    (default) -> sWarningOFF
    sWarningOFF -> sWarningON : [PwrSta == ENUM_POWERSTA_STANDBY && ...
        |  (VDDM_HVRlyOpCFS_flg || VDDM_MCUActCFS_flg)]
    sWarningON -> sWarningOFF : [PwrSta != ENUM_POWERSTA_STANDBY || ...
        |  (!VDDM_HVRlyOpCFS_flg && !VDDM_MCUActCFS_flg)]
  state Main [parallel]
    settings: executionOrder=3
    state sUnLockOFF1
      en:InputMode=0;
    state WelcomeOFF
      en:InputMode=0;
      WelcomeLight=0;
    state sWait
      en:LTurnLP=0;RTurnLP=0;
      WelcomeLight=0;
      BCMBuzzerReq=0;
    state sUnLockOFF
      en:LTurnLP=0;
      RTurnLP=0;
      FlashCount=FlashCount-1;
    state LockModeEND
      en:InputMode=0;
      WelcomeLight=0;
    state sLockOFF
      en:LTurnLP=0;
      RTurnLP=0;
      InputMode=0;
    state sHazardOFF
      en:LTurnLP=0;
      RTurnLP=0;
    state sESSOFF
      en:LTurnLP=0;
      RTurnLP=0;
    state sAlarmOFF
      en:LTurnLP=0;
      RTurnLP=0;
    note: 600 ms
    note: 500 ms
    state WelcomeMode
      en:WelcomeLight=1;
    note: 100 ms
    state sLock
      en:LTurnLP=1;
      RTurnLP=1;
    state LockMode
      en:WelcomeLight=2;
    state sUnlock
      en:LTurnLP=1;
      RTurnLP=1;
    note: 200 ms
    note: 500 ms
    note: 460 ms
    note: 460 ms
    note: 120 ms
    state sHazardON
      en:LTurnLP=1;
      RTurnLP=1;
    state sESSON
      en:LTurnLP=1;
      RTurnLP=1;
    state sAlarm
      en:LTurnLP=1;
      RTurnLP=1;
    state sOFF
      en:LTurnLP=0;RTurnLP=0;
    state TPMS
      en:
      LTurnLP = 1;
      RTurnLP = 1;
    state sLeftON
      en:LTurnLP=1;
      RTurnLP=0;
    state sRightON
      en:LTurnLP=0;
      RTurnLP=1;
    state sSPTG
      en:LTurnLP=1;
      RTurnLP=1;
      BCMBuzzerReq=1;
    state sRAPSAbnFlashON
      en:LTurnLP=1;
      RTurnLP=1;
    note: 230 ms
    note: 230 ms
    state sOFFNG
      en:LTurnLP=0;
      RTurnLP=0;
    note: 500 ms
    note: 500 ms
    state sSPTGOFF
      en:LTurnLP=0;
      RTurnLP=0;
      BCMBuzzerReq=0;
    state sRAPSAbnFlashOFF
      en:LTurnLP=0;
      RTurnLP=0;
    note: 230 ms
    note: 230 ms
    state sRightKeep
    state sLeftKeep
    note: 230 ms
    state sOFFOK
      en:LTurnLP=0;
      RTurnLP=0;
    Main -> sWait : [OutMode!=InputMode]
        | {OutMode=InputMode;}
    sUnLockOFF -> sUnLockOFF1 [order 1] : [FlashCount==0]
    WelcomeMode -> WelcomeOFF : [ !VBCM_UnlockWelcomeEN_flg ||....
        | after(KBCM_WelcomeT_s,tick) ]
    sLock -> sLockOFF : [after(50,tick)]
    LockMode -> LockModeEND : [after(KBCM_WelLockT_s,tick)]
    sUnlock -> sUnLockOFF : [after(20,tick)]
    sUnLockOFF -> sUnlock [order 2] : [after(60,tick)]
    sWait -> sOFF : [after(12,tick)]
    sAlarm -> sAlarmOFF : [after(50,tick)]
    sAlarmOFF -> sAlarm : [after(50,tick)]
    sHazardON -> sHazardOFF : [after(46,tick)]
    sHazardOFF -> sHazardON : [after(46,tick)]
    sESSON -> sESSOFF : [after(VBCM_ESSOnT_tick ,tick)]
    sESSOFF -> sESSON : [after(VBCM_ESSOffT_tick,tick)]
    (junction 2228) -> WelcomeMode
    (junction 2226) -> sUnlock [order 2] : {FlashCount=3;}
    sOFF -> sUnlock [order 1] : [InputMode==9]....
        | {FlashCount=2;}
    (junction 2132) -> sLock [order 2]
    (junction 2133) -> LockMode
    (default) -> sOFF
    sOFF -> sAlarm [order 8] : [OutMode==6]
    sOFF -> sHazardON [order 11] : [OutMode==3]
    sOFF -> sESSON [order 7] : [OutMode==7]
    (junction 2226) -> (junction 2228) [order 1] : [VBCM_UnlockWelcomeEN_flg]
    (junction 2132) -> (junction 2133) [order 1] : [VINP_VehicleType_enum == ENUM_VEHICLETYPE_D21]
    sOFF -> (junction 2226) [order 2] : [OutMode==5]
    sOFF -> (junction 2132) [order 3] : [OutMode==4]
    sOFF -> sSPTG [order 6] : [OutMode==8]
    sOFF -> sLeftON [order 9] : [OutMode==1]
    sOFF -> sRightON [order 10] : [OutMode==2]
    sOFF -> TPMS [order 5] : [OutMode == 11]
    sOFF -> sRAPSAbnFlashON [order 4] : [OutMode==12]
    (junction 1940) -> sLeftON [order 1] : [OutMode==1]
    (junction 1940) -> sRightON [order 2]
    sOFFNG -> (junction 1940) : [after(23,tick)]
    sLeftON -> (junction 1918) : [after(23,tick)]
    sRightON -> (junction 1929) : [after(23,tick)]
    sRAPSAbnFlashON -> sRAPSAbnFlashOFF : [after(KBCM_RAPSAbnFlashONT_ms,tick)]
    sRAPSAbnFlashOFF -> sRAPSAbnFlashON : [after(KBCM_RAPSAbnFlashOFFT_ms,tick)]
    sSPTG -> sSPTGOFF : [after(50,tick)]
    sSPTGOFF -> sSPTG : [after(50,tick)]
    (junction 2062) -> sOFFNG [order 1] : [FRTurnLPNormal]
        | {DiagFRTS=0;DiagRRTS=1;}
    (junction 1929) -> (junction 2062) [order 2]
    (junction 1918) -> (junction 2053) [order 2]
    (junction 2053) -> sOFFNG [order 1] : [FLTurnLPNormal]
        | {DiagFLTS=0;DiagRLTS=1;}
    (junction 2062) -> (junction 2065) [order 2]
    (junction 1929) -> sRightKeep [order 1] : [RRTurnLPNormal &&...
        | FRTurnLPNormal]
        | {DiagFRTS=0;DiagRRTS=0;}
    (junction 1918) -> sLeftKeep [order 1] : [RLTurnLPNormal &&...
        | FLTurnLPNormal]
        | {DiagFLTS=0;DiagRLTS=0;}
    (junction 2053) -> (junction 2056) [order 2]
    (junction 2056) -> sOFFNG [order 1] : [RLTurnLPNormal]
        | {DiagFLTS=1;DiagRLTS=0;}
    (junction 2065) -> sOFFNG [order 1] : [RRTurnLPNormal]
        | {DiagFRTS=1;DiagRRTS=0;}
    (junction 2056) -> (junction 2059) [order 2]
    (junction 2065) -> (junction 2068) [order 2]
    (junction 2059) -> sOFFNG : {DiagFLTS=1;DiagRLTS=1;}
    (junction 2068) -> sOFFNG : {DiagFRTS=1;DiagRRTS=1;}
    sOFFOK -> sOFFNG : [after(23,tick)]
    sRightKeep -> sOFFOK : [after(23,tick)]
    sLeftKeep -> sOFFOK : [after(23,tick)]
  data: ATCtrl input uint8 [0..2]; ATAlarm input boolean; PwrSta input uint8 [0..5]; HazardSWSta input boolean [0..1]; CSW_TurnSw_Sta input uint8 [0..3]; PTG_RDIL_Sta input; HazardSW output boolean =0; LTurnLP output boolean; RTurnLP output boolean; InputMode local uint8; FlashCount local uint8; OutMode output uint8; ESS_Active input boolean; LeftTurnLightReq input boolean; RightTurnLightReq input boolean; SPTGDet input boolean; HazardWarningReq input; DiagFLTS output; DiagFRTS output; DiagRLTS output; DiagRRTS output; BCMBuzzerReq output boolean; FALSE parameter; TRUE parameter; ENUM_POWERSTA_STANDBY parameter; VDDM_HVRlyOpCFS_flg input; VDDM_MCUActCFS_flg input; VBCM_PwrErrWarn_flg local boolean; VBCM_ESSOnT_tick input; VBCM_ESSOffT_tick input; VTPM_TPMSTLCmd_flg input; RLTurnLPNormal input; RRTurnLPNormal input; KBCM_WelcomeT_s input; KBCM_WelLockT_s input; VINP_VehicleType_enum input; FRTurnLPNormal input; FLTurnLPNormal input; VBCM_UnlockWelcomeEN_flg input; WelcomeLight output uint8; KBCM_RAPSAbnFlashOFFT_ms input; KBCM_RAPSAbnFlashONT_ms input; RAPSBCMLampCmd input; VBCM_RAPSAbnFlashReq_flg input; VINP_RAPSErrWarn_enum input; ENUM_VEHICLETYPE_D21 parameter

== stateflow chart bcm/BCM/BCM/PowerMirror/Chart ==
  settings: sampleTime=StepSize
  state sPowerFlag [parallel]
    settings: executionOrder=1
    state sActive
      en:PFlag=1;
    state sOff
      en:PFlag=0;
    state sDelay
      en:PFlag=1;
    (default) -> sOff
    sOff -> sActive : [PwrSta>3]
    sDelay -> sActive [order 1] : [PwrSta>3]
    sActive -> sDelay : [PwrSta<=3]
    (junction 1609) -> sOff
    sDelay -> (junction 1609) [order 2] : [after(3000,tick)]
  state sMirrorFoldSw [parallel]
    settings: executionOrder=2  description=This state models the modes of a door sensor and implements logic to respond when that sensor is producing a signal.
    state sRelease
    state sPush
      en:sMain.eMFSW;
    (default) -> sRelease
      settings: description=On the first sample call the door mode is set to active.
    sPush -> sRelease : [!MirrorFoldSw]
    sRelease -> sPush : [MirrorFoldSw]
  state sMain [parallel]
    settings: executionOrder=5
    state Close
      en:
      MirrorCtrl = 0;
      MirrorFlodPos = 0;
      MirrorFolderState = 0;
    state Mirror2Open
      en:
      MirrorCtrl = 2;
      MirrorFolderState = 1;
    state Suspend2Open
      en:
      MirrorCtrl = 0;
      MirrorFolderState = 4;
    state Suspend2Close
      en:
      MirrorCtrl = 0;
      MirrorFolderState = 5;
    state Mirror2Close
      en:
      MirrorCtrl = 1;
      MirrorFolderState = 3;
    state Open
      en:
      MirrorCtrl = 0;
      MirrorFlodPos = 1;
      MirrorFolderState = 2;
    (default) -> (junction 1709) : {MFSWTri=EEP_MFSWTri_flg;}
    (junction 1709) -> (junction 1710) [order 2]
    (junction 1709) -> Close [order 1] : [!EEP_MirrorFlodPos]{DisAntiTheftReq=EEP_MFSWTri_flg;}
    (junction 1710) -> Open
    Close -> (junction 1711) [order 1] : eMirrorUnlock[(PwrSta<=4&&!DisAntiTheftReq)||APS_Sta_System==4]
    (junction 1711) -> (junction 1712)
    Close -> (junction 1712) [order 2] : eMFSW[PFlag]/{DisAntiTheftReq=0;}
    (junction 1712) -> (junction 1713)
    Close -> (junction 1713) [order 3] : eAutoOpen/{DisAntiTheftReq=0;}
    (junction 1713) -> (junction 1765)
    Close -> (junction 1765) [order 4] : eCarWashUnfold
    (junction 1765) -> (junction 1770)
    Close -> (junction 1770) [order 5] : [IVIMirrorFoldedReq]
    (junction 1770) -> Mirror2Open
    Suspend2Open -> (junction 1770) [order 2] : [after(10,tick)]
    Mirror2Open -> Suspend2Close [order 1] : eMirrorLock
        | [PwrSta<=4||APS_Sta_System==4]/{MFSWTri=0;}
    Mirror2Open -> Suspend2Close [order 3] : eMFSW[PFlag]/{MFSWTri=1}
    Mirror2Open -> Suspend2Close [order 4] : eCarWashFold
    Mirror2Open -> Suspend2Close [order 5] : [IVIMirrorFoldedReq]
    Mirror2Open -> Open [order 2] : [after(600,tick)]
    Mirror2Close -> Close [order 2] : [after(600,tick)]/{DisAntiTheftReq=MFSWTri;}
    Mirror2Close -> Suspend2Open [order 3] : eMFSW[PFlag]
    Mirror2Close -> Suspend2Open [order 1] : eMirrorUnlock
        | [PwrSta<=4||APS_Sta_System==4]
    Mirror2Close -> Suspend2Open [order 4] : [IVIMirrorFoldedReq]
    Suspend2Open -> Suspend2Close [order 1] : eCarWashFold
    Suspend2Close -> (junction 1714) : [after(10,tick)]
    Open -> (junction 1714) [order 2] : eMFSW[PFlag]/{MFSWTri=1}
    (junction 1714) -> Mirror2Close
    (junction 1715) -> (junction 1714)
    Open -> (junction 1715) [order 1] : eMirrorLock[PwrSta<=4||APS_Sta_System==4]....
        | /{MFSWTri=0;}
    (junction 1782) -> (junction 1715)
    Open -> (junction 1782) [order 3] : [IVIMirrorFoldedReq]
    (junction 1786) -> (junction 1782)
    Open -> (junction 1786) [order 4] : eCarWashFold
  state sATCtrl [parallel]
    settings: executionOrder=4
    state StandBy
    state Lock
      en: sMain.eMirrorLock;
    state Unlock
      en: sMain.eMirrorUnlock;
    (default) -> sATCtrl.StandBy
    sATCtrl.StandBy -> Lock [order 1] : [ATActCtrl==1]
    Lock -> sATCtrl.StandBy : [ATActCtrl!=1]
    sATCtrl.StandBy -> Unlock [order 2] : [ATActCtrl==2]
    Unlock -> sATCtrl.StandBy : [ATActCtrl!=2]
  state sRemoteControl [parallel]
    settings: executionOrder=6
    state Standby
    state Fold
      en: sMain.eMirrorLock;
    state Unfold
      en: sMain.eMirrorUnlock;
    (default) -> Standby
    Standby -> Fold [order 1] : [VINP_ReOutsideMirror_enum == 1]
    Fold -> Standby : [VINP_ReOutsideMirror_enum != 1]
    Standby -> Unfold [order 2] : [VINP_ReOutsideMirror_enum == 2]
    Unfold -> Standby : [VINP_ReOutsideMirror_enum != 2]
  state sAutoOpen [parallel]
    settings: executionOrder=3
    state Reset
    state AutoOpenRequest
      en:sMain.eAutoOpen;
    (default) -> Reset
    Reset -> AutoOpenRequest : [VehSpeed>30 &&...
        | VehSpeed<256 &&...
        | PwrSta>3]
    AutoOpenRequest -> Reset : [PwrSta<=3]
  state CarWashMode [parallel]
    settings: executionOrder=7
    state StandBy
    state WaitForUnfold
    state AutoUnfoldDisable
    (default) -> CarWashMode.StandBy
    CarWashMode.StandBy -> WaitForUnfold : [hasChanged(IVICarWashModeCmd) && IVICarWashModeCmd == 1 && ....
        | (MirrorFolderState == 1 || MirrorFolderState == 2 || MirrorFolderState == 4)]
        | {send(eCarWashFold,sMain);}
    WaitForUnfold -> CarWashMode.StandBy [order 1] : [!IVICarWashModeCmd]{send(eCarWashUnfold,sMain);}
    WaitForUnfold -> AutoUnfoldDisable [order 2] : [hasChanged(MirrorCtrl) && MirrorCtrl == 2]
    AutoUnfoldDisable -> CarWashMode.StandBy : [!IVICarWashModeCmd]
  data: PwrSta input uint8 [0..4]; MirrorFoldSw input boolean; VehSpeed input [0..4096]; MirrorCtrl output uint8 [0..2] =0; PFlag local boolean; DisAntiTheftReq local boolean =0; ATActCtrl input uint8 [0..2]; VINP_ReOutsideMirror_enum input; MFSWTri output boolean =0; EEP_MFSWTri_flg input; MirrorFlodPos output; EEP_MirrorFlodPos input; APS_Sta_System input; IVICarWashModeCmd input; MirrorFolderState local uint8; IVIMirrorFoldedReq input
  data VehSpeed settings: description=Min=0, Max=2047, Engineering Unit = km/h, Offset=0 km/h, Resolution= 0.125 km/h per bit, >2047 = Invalid (bit 12 = 1)
  data MirrorCtrl settings: description=|
      | Bcm Buzzer output results.
      | 0 = None Buzzer
      | 1 = Turn signal Buzzer
      | 2 = Key Reminder Buzzer
      | 3 = Seat Belt Buzzer
      | 4 = Light Monitor Buzzer
  events: eAutoOpen local EITHER_EDGE_EVENT; eMFSW local EITHER_EDGE_EVENT; eMirrorUnlock local FUNCTION_CALL_EVENT; eMirrorLock local FUNCTION_CALL_EVENT; eCarWashFold local FUNCTION_CALL_EVENT; eCarWashUnfold local FUNCTION_CALL_EVENT

== stateflow chart bcm/BCM/BCM/RearDefogger/Chart ==
  settings: sampleTime=StepSize
  state CANCMD [parallel]
    settings: executionOrder=1
    state OFF
    state StandBy
    state Press
    (default) -> OFF
    OFF -> StandBy : [PwrSta>3]
    StandBy -> OFF [order 1] : [PwrSta<=3]
    StandBy -> Press [order 2] : [RR_Def_Sta||IVI_RR_Def_Req]{sMain.eRRDefPress;}
    Press -> StandBy [order 2] : [!RR_Def_Sta&&!IVI_RR_Def_Req]
    Press -> OFF [order 1] : [PwrSta<=3]
  state sMain [parallel]
    settings: executionOrder=2  description=This state models the modes of a door sensor and implements logic to respond when that sensor is producing a signal.
    state sOFF
      en:MirrorDefog=0;
      RearDefog=0;
    state sON
      en:MirrorDefog=1;
      RearDefog=1;
    note: 20 min
    (default) -> sOFF
      settings: description=On the first sample call the door mode is set to active.
    sOFF -> sON : eRRDefPress
    sON -> sOFF [order 1] : [PwrSta<=3]
    sON -> sOFF [order 2] : [after(120000,tick)]
    sON -> sOFF [order 3] : eRRDefPress
  data: PwrSta input uint8 [0..4]; RR_Def_Sta input boolean; IVI_RR_Def_Req input boolean; MirrorDefog output boolean =0; RearDefog output boolean
  data IVI_RR_Def_Req settings: description=Min=0, Max=2047, Engineering Unit = km/h, Offset=0 km/h, Resolution= 0.125 km/h per bit, >2047 = Invalid (bit 12 = 1)
  data MirrorDefog settings: description=|
      | Bcm Buzzer output results.
      | 0 = None Buzzer
      | 1 = Turn signal Buzzer
      | 2 = Key Reminder Buzzer
      | 3 = Seat Belt Buzzer
      | 4 = Light Monitor Buzzer
  events: eRRDefPress local FUNCTION_CALL_EVENT

== stateflow chart bcm/BCM/BCM/RoomLamp/Chart ==
  settings: sampleTime=StepSize
  state sDoorLockSta [parallel]
    settings: executionOrder=1  description=This state models the modes of a door sensor and implements logic to respond when that sensor is producing a signal.
    state sLock
    state sUnlock
    (default) -> (junction 1595)
    (junction 1595) -> sUnlock [order 2]
    (junction 1595) -> sLock [order 1] : [DrLockSW]
    sLock -> sUnlock : [DrLockSW==0]/sMain.eDrDoorUnlock
    sUnlock -> sLock : [DrLockSW==1]/sMain.eDrDoorLock
  state sRoomLampPower [parallel]
    settings: executionOrder=2
    state sON
      note: 40min
      state Keep
        en:
        RoomLampH=1;
        RoomLampTmr=0;
      state KeyIn
        en:
        RoomLampTmr=RoomLampTmr+task_time_s;
        du:
        RoomLampTmr=RoomLampTmr+task_time_s;
      state KeyMiss
        en:
        RoomLampTmr=RoomLampTmr+task_time_s;
        du:
        RoomLampTmr=RoomLampTmr+task_time_s;
      note: 10min
      (default) -> Keep
      Keep -> KeyIn [order 1] : [P_DKey_Area_LockUnlock==ENUM_PDKEYRAWLULOCK_INUNLOCK && ...
          |  P_DKey_Area_PS != ENUM_PDKEYRAWPS_INPS && ...
          |  PwrSta<4]
      KeyIn -> (junction 1756) [order 1] : [RoomLampTmr>=KBCM_RmLpKeyInT_s]
      (junction 1756) -> (junction 1760)
      KeyIn -> Keep [order 2] : [DoorOpen || PwrSta>3 || ...
          |  P_DKey_Area_PS==ENUM_PDKEYRAWPS_INPS]
      KeyMiss -> KeyIn [order 3] : [P_DKey_Area_LockUnlock==ENUM_PDKEYRAWLULOCK_INUNLOCK]
      KeyIn -> KeyMiss [order 3] : [P_DKey_Area_LockUnlock!=ENUM_PDKEYRAWLULOCK_INUNLOCK]
      KeyMiss -> Keep [order 2] : [DoorOpen || PwrSta>3 || ...
          |  P_DKey_Area_PS==ENUM_PDKEYRAWPS_INPS]
      KeyMiss -> (junction 1760) [order 1] : [RoomLampTmr>=KBCM_RmLpKeyMissT_s]
      Keep -> KeyMiss [order 2] : [P_DKey_Area_LockUnlock!=ENUM_PDKEYRAWLULOCK_INUNLOCK && ...
          |  P_DKey_Area_PS!=ENUM_PDKEYRAWPS_INPS && ...
          |  PwrSta<4]
    state sKeyON
      state sOFF
        en:RoomLampH=0;
      state sSAVEPower
        en:RoomLampH=0;
      state sKeep
        en:RoomLampH=1;
      sKeep -> sRoomLampPower.sKeyON.sOFF [order 2] : [AntitheftSta==1||AntitheftSta==3]
      sSAVEPower -> sRoomLampPower.sKeyON.sOFF : [AntitheftSta==1||AntitheftSta==3]
      (default) -> sSAVEPower
      sKeep -> sSAVEPower [order 1] : [after(KBCM_RmLampKeep_min,tick)]
    (default) -> sKeyON
    sRoomLampPower.sKeyON.sOFF -> sRoomLampPower.sON : [AntitheftSta==0||AntitheftSta==2]
    sKeyON -> sRoomLampPower.sON : [PwrSta>3||DoorOpen]
    sRoomLampPower.sON -> sKeep : [PwrSta<4&&!AllDoorSW&&!TailgateSW]
    (junction 1760) -> sSAVEPower
  state sMain [parallel]
    settings: executionOrder=3
    state sFunctionOFF
      en:RoomLampL=0;
    state sLampOFF
      state sOFF
        en:RoomLampL=0;
      state sKEEP
        en:RoomLampL=1;
      (junction 1665) -> sMain.sLampOFF.sOFF : [after(3000,tick)||....
          | (PwrSta==ENUM_PWRSTASW_ON....
          | ||....
          | PwrSta==ENUM_PWRSTASW_READY)]
      (junction 1666) -> sMain.sLampOFF.sOFF [order 2] : eDrDoorLock
      sMain.sLampOFF.sOFF -> sKEEP : eDrDoorUnlock
          | [PwrSta!=ENUM_PWRSTASW_ON....
          | &&....
          | PwrSta!=ENUM_PWRSTASW_READY]
      (junction 1666) -> (junction 1665) [order 1]
      sKEEP -> (junction 1666)
    state sON
      en:RoomLampL=1;
    (default) -> sFunctionOFF
    sFunctionOFF -> sMain.sLampOFF.sOFF : [FDC_BCM_RmLpModeENFun_Sta==1]
    sLampOFF -> sFunctionOFF [order 1] : [FDC_BCM_RmLpModeENFun_Sta==0]
    sMain.sON -> sFunctionOFF [order 1] : [FDC_BCM_RmLpModeENFun_Sta==0]
    (junction 1653) -> sMain.sLampOFF.sOFF
    (junction 1652) -> sKEEP [order 2]
    sLampOFF -> sMain.sON [order 2] : [AllDoorSW]
    (junction 1652) -> (junction 1653) [order 1] : [PwrSta==ENUM_PWRSTASW_ON....
        | ||....
        | PwrSta==ENUM_PWRSTASW_READY]
    sMain.sON -> (junction 1652) [order 2] : [AllDoorSW==0]
  data: task_time_s input single; PwrSta input uint8 [0..5]; RoomLampH output boolean =0; DrLockSW input boolean; AllDoorSW input boolean; DoorOpen input boolean; RoomLampL output boolean =0; AntitheftSta input uint8 [0..3]; TailgateSW input boolean; KBCM_RmLampKeep_min input; FDC_BCM_RmLpModeENFun_Sta input boolean =0; RoomLampTmr output single =0; P_DKey_Area_LockUnlock input uint8; P_DKey_Area_PS input uint8; KBCM_RmLpKeyInT_s input; KBCM_RmLpKeyMissT_s input; ENUM_PDKEYRAWPS_INPS parameter; ENUM_PDKEYRAWLULOCK_INUNLOCK parameter; ENUM_PWRSTASW_ON parameter; ENUM_PWRSTASW_READY parameter
  data RoomLampH settings: description=|
      | Bcm Buzzer output results.
      | 0 = None Buzzer
      | 1 = Turn signal Buzzer
      | 2 = Key Reminder Buzzer
      | 3 = Seat Belt Buzzer
      | 4 = Light Monitor Buzzer
  data DrLockSW settings: description=|
      | Door Lock Status
      | Lock =1
      | Unlock=0
  data RoomLampL settings: description=|
      | Bcm Buzzer output results.
      | 0 = None Buzzer
      | 1 = Turn signal Buzzer
      | 2 = Key Reminder Buzzer
      | 3 = Seat Belt Buzzer
      | 4 = Light Monitor Buzzer
  data AntitheftSta settings: description=|
      | 0 = Disarm Status
      | 1 = Arm Status
      | 2 = Wait for Rearm Status
      | 3 = Alarm Status
  events: eDrDoorLock local EITHER_EDGE_EVENT; eDrDoorUnlock local EITHER_EDGE_EVENT

== stateflow chart bcm/BCM/BCM/Tailgate/Chart ==
  settings: sampleTime=StepSize
  state TrunkRelease [parallel]
    settings: executionOrder=1
    state sStandBy
      en:TrunkRelease=0;
    state sDebounce
    state sUnlatch
      en:TrunkRelease=1;
    state sWaitForRelease
      en:TrunkRelease=0;
    (default) -> sStandBy
    sStandBy -> sDebounce : [TrunkHanSW==1]
    sDebounce -> (junction 1688) [order 1] : [after(20,tick)]
    (junction 1688) -> sUnlatch [order 1] : [!DrLockSta&&(PwrSta<=3||VehSpeed<5)]
    (junction 1688) -> sWaitForRelease [order 2]
    sDebounce -> sStandBy [order 2] : [TrunkHanSW==0]
    sUnlatch -> sWaitForRelease : [after(75,tick)]
    sWaitForRelease -> sStandBy : [TrunkHanSW==0]
  data: PwrSta input uint8 [0..4]; VehSpeed input [0..4047]; DrLockSta input boolean; TrunkRelease output boolean; TrunkHanSW input boolean
  data DrLockSta settings: description=Min=0, Max=2047, Engineering Unit = km/h, Offset=0 km/h, Resolution= 0.125 km/h per bit, >2047 = Invalid (bit 12 = 1)
